simulink model "rosio2"  (R2015a)
settings: Solver=ode3  StartTime=0.0  StopTime=inf  FixedStep=0.01  RelTol=1e-3
libraries: robotlib x2
settings Model: Creator=corkep  LastModifiedBy=corkep

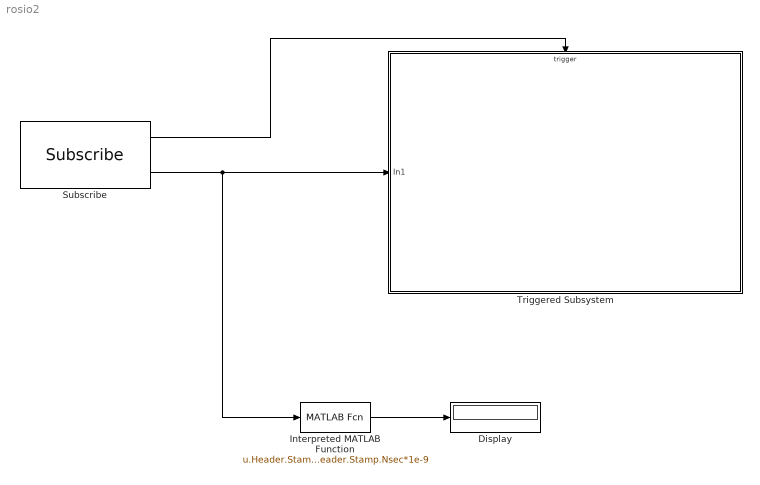
== system rosio2 ==
  Display : Display
  Interpreted MATLAB Function : MATLABFcn  MATLABFcn=u.Header.Stamp.Sec + u.Header.Stamp.Nsec*1e-9
  Subscribe : robotlib/Subscribe  SourceLibraryInfo=This block requires Robotics System Toolbox  topicSource=Specify your own  topic=/MyTopic4  messageType=geometry_msgs/TwistStamped  sampleTime=-1  messageQueueLength=1
  Triggered Subsystem : Subsystem  TreatAsAtomicUnit=on
  wires:
  Subscribe/2 -> Interpreted MATLAB Function/1, Triggered Subsystem/1(In1)
  Subscribe/1 -> Triggered Subsystem/Trigger
  Interpreted MATLAB Function/1 -> Display/1

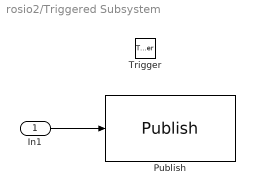
== system rosio2/Triggered Subsystem ==
  In1 : Inport
  Trigger : TriggerPort
  Publish : robotlib/Publish  SourceLibraryInfo=This block requires Robotics System Toolbox  topicSource=Specify your own  topic=/MyTopic  messageType=std_msgs/String  messageQueueLength=1
  wires:
  In1/1 -> Publish/1
